simulink model "v2_Ident_Planta"  (R2026a)
settings: Solver=FixedStepDiscrete  StopTime=inf  FixedStep=0.01  EnableMultiTasking=on
libraries: arduinolib x3, simulink x1, arduinosensorlib x1
settings Model: SILPILModeSetting=veronly  ExtModeTrigDuration=2  Creator=Lenovo  LastModifiedBy=Lenovo
settings HardwareCC: ProdLargestAtomicInteger=Long  ProdLargestAtomicFloat=Double  ProdHWDeviceType=ARM Compatible->ARM Cortex
settings RTWCC: SystemTargetFile=ert.tlc  HardwareBoard=ESP32-WROOM (Arduino Compatible)  TLCOptions="-aInlineSetEventsForThisBaseRateFcn=TLC_FALSE -aSuppressMultiTaskScheduler=TLC_FALSE  -aRateBasedStepFcn=0"  Toolchain=ESP32  BuildConfiguration=Faster Runs  Description=Embedded Coder
settings ERTTargetCC: ExtModeTransport=3.0  ExtModeAutomaticAllocSize=off  ExtModeStaticAllocSize=65536.0  RootIOFormat=Structure reference  SupportContinuousTime=on  SupportVariableSizeSignals=on

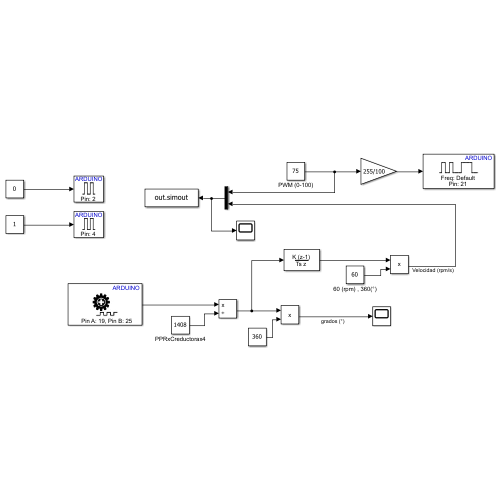
[thumbnail: Simulink's stored preview of the top-level diagram]
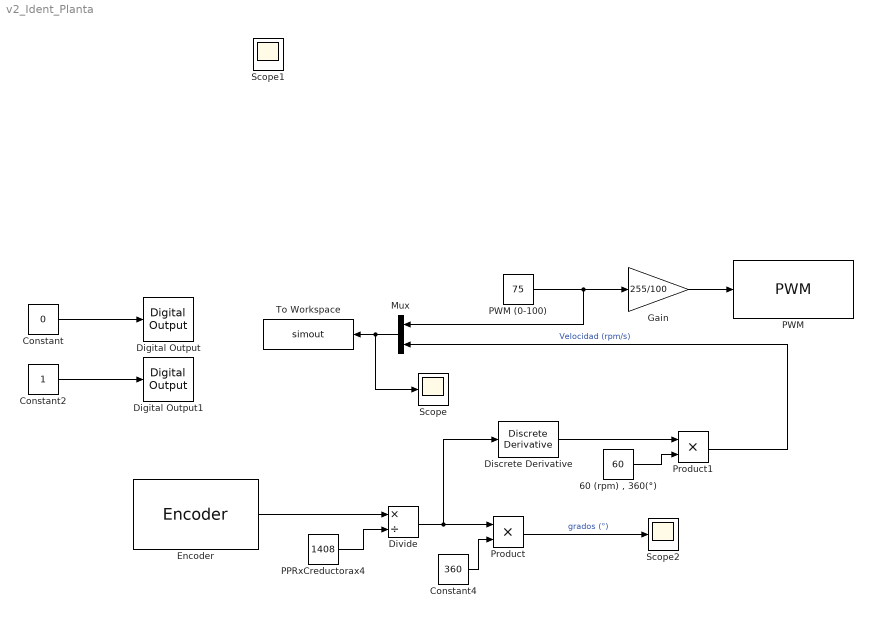
== system v2_Ident_Planta ==
  "60 (rpm) , 360(°)" : Constant  Value=60
  Constant : Constant  Value=0
  Constant2 : Constant
  Constant4 : Constant  Value=360
  Digital Output : arduinolib/Digital Output  pinNumber=2  Direction=output  blockPlatform=arduino
  Digital Output1 : arduinolib/Digital Output  pinNumber=4  Direction=output  blockPlatform=arduino
  Discrete Derivative : simulink/Discrete/Discrete Derivative  gainval=1.0  ICPrevScaledInput=0.0  OutMin=[]  OutMax=[]  OutDataType=fixdt(1, 16)  OutScaling=2^-10  DoSatur=off
  Divide : Product  Inputs=*/
  Encoder : arduinosensorlib/Encoder  InputA=19  InputB=25  Mode=No reset  SampleTime=-1
  Gain : Gain  Gain=255/100
  Mux : Mux  Inputs=2
  PPRxCreductorax4 : Constant  Value=1408
  PWM : arduinolib/PWM  pinNumber=21  frequencyType=Default  desiredFrequency=490.2  achievableFrequency=490.2
  PWM (0-100) : Constant  Value=75
  Product : Product
  Product1 : Product
  Scope : Scope
      settings: ActiveDisplayYMinimum=57.058540746019688  ActiveDisplayYMaximum=164.35261922617639
  Scope2 : Scope
      settings: ActiveDisplayYMinimum=-5504.7975852272721  ActiveDisplayYMaximum=49543.178267045456  DataLoggingVariableName=ScopeData2
  To Workspace : ToWorkspace  VariableName=simout  SaveFormat=Structure With Time  SampleTime=-1
  Scope1 : Scope
  wires:
  Constant2/1 -> Digital Output1/1
  PWM (0-100)/1 -> Mux/1, Gain/1
  Constant/1 -> Digital Output/1
  Mux/1 -> Scope/1, To Workspace/1
  Encoder/1 -> Divide/1
  PPRxCreductorax4/1 -> Divide/2
  Divide/1 -> Discrete Derivative/1, Product/1
  Constant4/1 -> Product/2
  Product/1 -> Scope2/1  "grados (°)"
  Discrete Derivative/1 -> Product1/1
  "60 (rpm) , 360(°)"/1 -> Product1/2
  Product1/1 -> Mux/2  "Velocidad (rpm/s)"
  Gain/1 -> PWM/1
